simulink model "s1c"  (Simulink 2.00)
settings: Solver=ode113  StartTime=0.0  StopTime=tstop  MaxStep=1e-2  RelTol=1e-5  AbsTol=1e-6
values from neighbouring files (symbols this model uses):
  Domega = 0    [P20HP.M]
  H = J*wbm*wbm/(2*Sb)    (= 3.33396824273)    [P20HP.M]
  Psidso = 0    [M1C.M]    (also in M1O.M; M3.M)
  Psipdro = 0    [M1C.M]    (also in M1O.M; M3.M)
  Psipqro = 0    [M1C.M]    (also in M1O.M; M3.M)
  Psiqso = 0    [M1C.M]    (also in M1O.M; M3.M)
  rpr = 0.0764    [P20HP.M]
  rs = 0.1062    [P20HP.M]
  smaxt = rpr/rpr1    [M1C.M]    (also in M1O.M)
  speed_wref = [0 0.5 0.5 -0.5 -0.5 0]    [M1C.M]    (also in M1O.M = [0 1 1]; M3.M = [0 wbm/2 wbm/2 -wbm/2 -wbm/2 0])
  Tfactor = (3*P)/(4*wb)    (= 0.00795774715459)    [P20HP.M]
  time_tmech = [0 4]    [M1C.M]    (also in M1O.M = [0 0.75 0.75 1.0 1.0 1.25 1.25 1.5 1.5 2]; M3.M = [0 tstop])
  time_wref = [0 0.25 0.5 1.0 1.25 1.5]    [M1C.M]    (also in M1O.M = [0 0.5 4]; M3.M)
  tmech_tmech = [0 0]    [M1C.M]    (also in M1O.M = [0 0 -Trated -Trated -Trated/2 -Trated/2 -Trated -Trated 0 0; M3.M)
  vrms_vf = vrms    [M1C.M]    (also in M1O.M)
  wb = 2*pi*frated    (= 376.991118431)    [P20HP.M]
  we_vf = w    [M1C.M]    (also in M1O.M)
  wrbywbo = 0    [M1C.M]    (also in M1O.M; M3.M)
  xls = (we/wb)*xls    [M1C.M]    (also in M1O.M; M3.M; P20HP.M = 0.2145)
  xM = 1/(1/xm + 1/xls + 1/xplr)    [M1C.M]    (also in M1O.M; M3.M; P20HP.M = 0.105313916498)
  xplr = (we/wb)*xplr    [M1C.M]    (also in M1O.M; M3.M; P20HP.M = 0.2145)
  Zb = Vrated*Vrated/Sb    (= 3.24396782842)    [P20HP.M]
settings Model: MaxOrder=3  SaveTime=off  SaveOutput=off  ConsistencyChecking=off

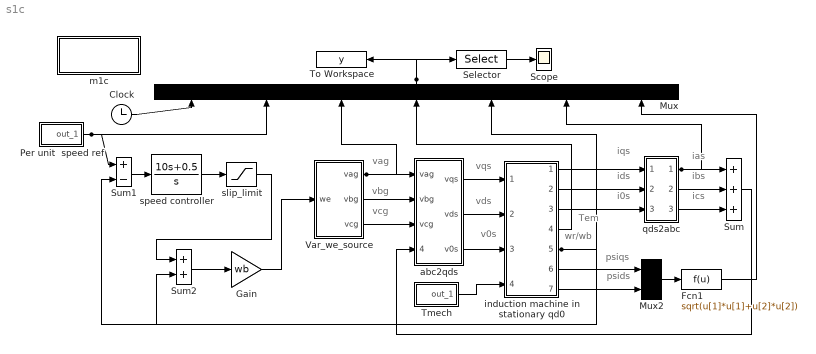
== system s1c ==
  note: wr/wb
  note: vcg
  note: vbg
  note: vag
  note: v0s
  note: vqs
  note: vds
  note: psiqs
  note: psids
  note: Tem
  note: i0s
  note: iqs
  note: ids
  note: ibs
  note: ias
  note: ics
  Clock : Clock
      settings: DeleteFcn=simclock BlockIsBeingDestroyed  PostSaveFcn=simclock Save
  Fcn1 : Fcn  Expr=sqrt(u[1]*u[1]+u[2]*u[2])
  Gain : Gain  Gain=wb
  m1c : Subsystem
      settings: OpenFcn=m1c
      mask Type: Masked block of m1c.m
      mask Help: Uses m1c.m to initialize and plot
      mask Display: disp('Initialize\nand plot')
  Mux : Mux  Orientation=up  Inputs=7
  Mux2 : Mux  Inputs=2
  "Per unit  speed ref " : Subsystem  mask(Repeating table){rep_seq_t=time_wref, rep_seq_y=speed_wref}
      mask prompts: rep_seq_t "Time values:"; rep_seq_y "Output values:"
      mask help: Repeating table.
      mask init:
      | period = max(rep_seq_t);
      mask Help: Repeats cycle given in table. Time values should be monotonically increasing.
      mask Display: plot([rep_seq_t,rep_seq_t+period,rep_seq_t+2*period,rep_seq_t(1)+3*period],[rep_seq_y,rep_seq_y,rep_seq_y,rep_seq_y(1)])
  Scope : Scope
      settings: TickLabels=on  TimeRange=2  YMin=-300  YMax=300  SaveToWorkspace=off  SaveName=ScopeData  LimitMaxRows=off
  Selector : Selector  Elements=[2 3 4 5 6 7]  InputPortWidth=7
  Sum : Sum  Inputs=+++
  Sum1 : Sum  Inputs=+-
  Sum2 : Sum  Inputs=++
  Tmech : Subsystem  mask(Repeating table){rep_seq_t=time_tmech, rep_seq_y=tmech_tmech}
      mask prompts: rep_seq_t "Time values:"; rep_seq_y "Output values:"
      mask help: Repeating table.
      mask init:
      | period = max(rep_seq_t);
      mask Help: Repeats cycle given in table. Time values should be monotonically increasing.
      mask Display: plot([rep_seq_t,rep_seq_t+period,rep_seq_t+2*period,rep_seq_t(1)+3*period],[rep_seq_y,rep_seq_y,rep_seq_y,rep_seq_y(1)])
  To Workspace : ToWorkspace  VariableName=y  SampleTime=0
      settings: Buffer=40000
  Var_we_source : Subsystem
  abc2qds : Subsystem
  induction machine in stationary qd0 : Subsystem
  qds2abc : Subsystem
  slip_limit : Saturate  UpperLimit=0.7*smaxt  LowerLimit=-0.7*smaxt
  speed controller : TransferFcn  Numerator=[10 0.5]  Denominator=[1 0]
  wires:
  abc2qds/3(v0s) -> induction machine in stationary qd0/3(in_v0s)
  Gain/1 -> Var_we_source/1(we)
  slip_limit/1 -> Sum2/1
  qds2abc/1(ias) -> Mux/6, Sum/1
  induction machine in stationary qd0/4(out_Tem) -> Mux/4
  Tmech/1(out_1) -> induction machine in stationary qd0/4(in_Tmech)
  Fcn1/1 -> Mux/7
  Var_we_source/1(vag) -> Mux/3, abc2qds/1(vag)
  "Per unit  speed ref "/1(out_1) -> Mux/2, Sum1/1
  Mux2/1 -> Fcn1/1
  induction machine in stationary qd0/7(out_psids) -> Mux2/2
  induction machine in stationary qd0/6(out_psiqs) -> Mux2/1
  speed controller/1 -> slip_limit/1
  induction machine in stationary qd0/5(out_wr/wb) -> Mux/5, Sum2/2, Sum1/2
  Sum2/1 -> Gain/1
  Sum1/1 -> speed controller/1
  induction machine in stationary qd0/3(out_i0s) -> qds2abc/3(i0s)
  induction machine in stationary qd0/2(out_ids) -> qds2abc/2(ids)
  induction machine in stationary qd0/1(out_iqs) -> qds2abc/1(iqs)
  abc2qds/2(vds) -> induction machine in stationary qd0/2(in_vds)
  Sum/1 -> abc2qds/4(ias+ibs+ics)
  qds2abc/3(ics) -> Sum/3
  qds2abc/2(ibs) -> Sum/2
  Var_we_source/3(vcg) -> abc2qds/3(vcg)
  Var_we_source/2(vbg) -> abc2qds/2(vbg)
  Clock/1 -> Mux/1
  abc2qds/1(vqs) -> induction machine in stationary qd0/1(in_vqs)
  Selector/1 -> Scope/1
  Mux/1 -> To Workspace/1, Selector/1

== system s1c/m1c ==
  note: Masked block of m1c.m
      | to initilialize simulation s1c.m
      | and to plot the results.

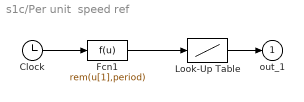
== system s1c/Per unit  speed ref  ==
  Clock : Clock
      settings: DeleteFcn=simclock BlockIsBeingDestroyed  PostSaveFcn=simclock Save
  Fcn1 : Fcn  Expr=rem(u[1],period)
  Look-Up Table : Lookup  InputValues=rep_seq_t  OutputValues=rep_seq_y
  out_1 : Outport  Port=1  InitialOutput=0
  wires:
  Fcn1/1 -> Look-Up Table/1
  Clock/1 -> Fcn1/1
  Look-Up Table/1 -> out_1/1

== system s1c/Tmech ==
  Clock : Clock
      settings: DeleteFcn=simclock BlockIsBeingDestroyed  PostSaveFcn=simclock Save
  Fcn1 : Fcn  Expr=rem(u[1],period)
  Look-Up Table : Lookup  InputValues=rep_seq_t  OutputValues=rep_seq_y
  out_1 : Outport  Port=1  InitialOutput=0
  wires:
  Fcn1/1 -> Look-Up Table/1
  Clock/1 -> Fcn1/1
  Look-Up Table/1 -> out_1/1

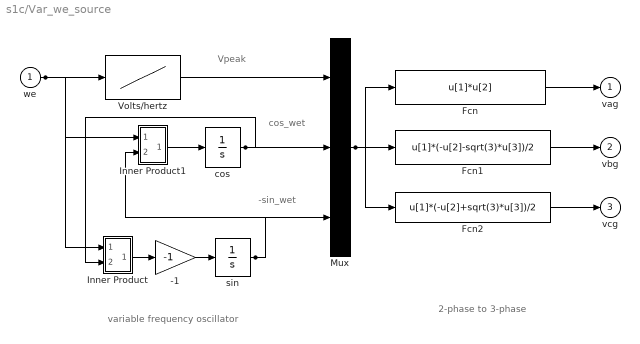
== system s1c/Var_we_source ==
  note: -sin_wet
  note: cos_wet
  note: variable frequency oscillator
  note: 2-phase to 3-phase
  note: Vpeak
  we : Inport  Port=1  PortWidth=-1  SampleTime=-1
  -1 : Gain  Gain=-1
  Fcn : Fcn  Expr=u[1]*u[2]
  Fcn1 : Fcn  Expr=u[1]*(-u[2]-sqrt(3)*u[3])/2
  Fcn2 : Fcn  Expr=u[1]*(-u[2]+sqrt(3)*u[3])/2
  Inner Product : Subsystem
      mask Type: Dot Product
      mask Description:
      | Inner (dot) product.
      | y=sum(u1.*u2)
      mask Help: Computes the inner (dot) product of the inputs: sum(u1.*u2).  The inputs are vectors of the same length. Output is a scalar.
      mask Display: disp('.\n')
  Inner Product1 : Subsystem
      mask Type: Dot Product
      mask Description:
      | Inner (dot) product.
      | y=sum(u1.*u2)
      mask Help: Computes the inner (dot) product of the inputs: sum(u1.*u2).  The inputs are vectors of the same length. Output is a scalar.
      mask Display: disp('.\n')
  Mux : Mux  Inputs=3
  Volts/hertz : Lookup  InputValues=we_vf  OutputValues=vrms_vf
  cos : Integrator  ExternalReset=none  InitialConditionSource=internal  InitialCondition=1  LimitOutput=off  UpperSaturationLimit=inf  LowerSaturationLimit=-inf  ShowSaturationPort=off  ShowStatePort=off  AbsoluteTolerance=auto
  sin : Integrator  ExternalReset=none  InitialConditionSource=internal  InitialCondition=0  LimitOutput=off  UpperSaturationLimit=inf  LowerSaturationLimit=-inf  ShowSaturationPort=off  ShowStatePort=off  AbsoluteTolerance=auto
  vag : Outport  Port=1  InitialOutput=0
  vbg : Outport  Port=2  InitialOutput=0
  vcg : Outport  Port=3  InitialOutput=0
  wires:
  Volts/hertz/1 -> Mux/1
  we/1 -> Volts/hertz/1, Inner Product/1(in_1), Inner Product1/1(in_1)
  Mux/1 -> Fcn2/1, Fcn1/1, Fcn/1
  Fcn2/1 -> vcg/1
  Fcn1/1 -> vbg/1
  Fcn/1 -> vag/1
  sin/1 -> Mux/3, Inner Product1/2(in_2)
  cos/1 -> Mux/2, Inner Product/2(in_2)
  Inner Product1/1(out_1) -> cos/1
  Inner Product/1(out_1) -> -1/1
  -1/1 -> sin/1

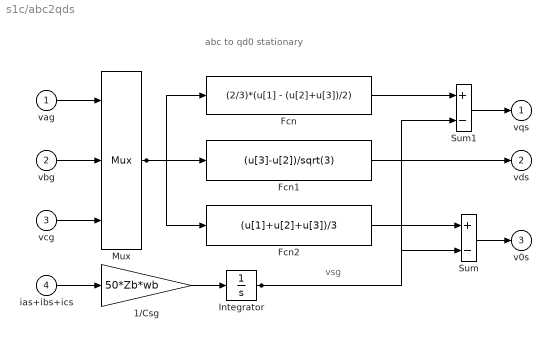
== system s1c/abc2qds ==
  note: vsg
  note: abc to qd0 stationary
  vag : Inport  Port=1  PortWidth=-1  SampleTime=-1
  vbg : Inport  Port=2  PortWidth=-1  SampleTime=-1
  vcg : Inport  Port=3  PortWidth=-1  SampleTime=-1
  ias+ibs+ics : Inport  Port=4  PortWidth=-1  SampleTime=-1
  1/Csg : Gain  Gain=50*Zb*wb
  Fcn : Fcn  Expr=(2/3)*(u[1] - (u[2]+u[3])/2)
  Fcn1 : Fcn  Expr=(u[3]-u[2])/sqrt(3)
  Fcn2 : Fcn  Expr=(u[1]+u[2]+u[3])/3
  Integrator : Integrator  ExternalReset=none  InitialConditionSource=internal  InitialCondition=0  LimitOutput=off  UpperSaturationLimit=inf  LowerSaturationLimit=-inf  ShowSaturationPort=off  ShowStatePort=off  AbsoluteTolerance=auto
  Mux : Mux  Inputs=3
  Sum : Sum  Inputs=+-
  Sum1 : Sum  Inputs=+-
  vqs : Outport  Port=1  InitialOutput=0
  vds : Outport  Port=2  InitialOutput=0
  v0s : Outport  Port=3  InitialOutput=0
  wires:
  Integrator/1 -> Sum1/2, Sum/2
  Sum1/1 -> vqs/1
  Fcn/1 -> Sum1/1
  1/Csg/1 -> Integrator/1
  Fcn2/1 -> Sum/1
  Sum/1 -> v0s/1
  Fcn1/1 -> vds/1
  Mux/1 -> Fcn2/1, Fcn/1, Fcn1/1
  vcg/1 -> Mux/3
  vbg/1 -> Mux/2
  vag/1 -> Mux/1
  ias+ibs+ics/1 -> 1/Csg/1

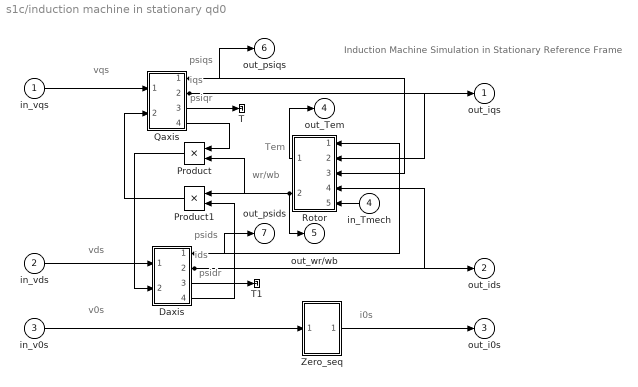
== system s1c/induction machine in stationary qd0 ==
  note: psiqs
  note: psids
  note: v0s
  note: i0s
  note: Tem
  note: wr/wb
  note: vds
  note: vqs
  note: ids
  note: psidr
  note: psiqr
  note: iqs
  note: Induction Machine Simulation
      |   in Stationary Reference Frame
  in_vqs : Inport  Port=1  PortWidth=-1  SampleTime=-1
  in_vds : Inport  Port=2  PortWidth=-1  SampleTime=-1
  in_v0s : Inport  Port=3  PortWidth=-1  SampleTime=-1
  in_Tmech : Inport  Orientation=left  Port=4  PortWidth=-1  SampleTime=-1
  Daxis : Subsystem
  Product : Product  Orientation=left  Inputs=2
  Product1 : Product  Orientation=left  Inputs=2
  Qaxis : Subsystem
  Rotor : Subsystem  Orientation=left
  T : Terminator
  T1 : Terminator
  Zero_seq : Subsystem
  out_iqs : Outport  Port=1  InitialOutput=0
  out_ids : Outport  Port=2  InitialOutput=0
  out_i0s : Outport  Port=3  InitialOutput=0
  out_Tem : Outport  Port=4  InitialOutput=0
  out_wr/wb : Outport  Port=5  InitialOutput=0
  out_psiqs : Outport  Port=6  InitialOutput=0
  out_psids : Outport  Port=7  InitialOutput=0
  wires:
  Daxis/3(out_idr') -> T1/1
  Qaxis/3(out_iqr') -> T/1
  Daxis/1(out_psids) -> out_psids/1, Rotor/1(in_psids)
  Qaxis/1(out_psiqs) -> out_psiqs/1, Rotor/3(in_psiqs)
  Daxis/2(out_ids) -> out_ids/1, Rotor/4(in_ids)
  Qaxis/2(out_iqs) -> out_iqs/1, Rotor/2(in_iqs)
  Zero_seq/1(out_i0s) -> out_i0s/1
  in_vds/1 -> Daxis/1(in_vds)
  in_v0s/1 -> Zero_seq/1(in_v0s)
  in_vqs/1 -> Qaxis/1(in_vqs)
  in_Tmech/1 -> Rotor/5(in_Tmech)
  Rotor/1(out_Tem) -> out_Tem/1
  Product1/1 -> Qaxis/2(in_(wr/wb)*psidr')
  Product/1 -> Daxis/2(in_(wr/wb)*psiqr')
  Rotor/2(out_wr/wb) -> out_wr/wb/1, Product/2, Product1/1
  Qaxis/4(out_psiqr') -> Product/1
  Daxis/4(out_psidr') -> Product1/2

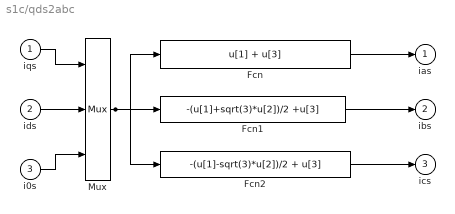
== system s1c/qds2abc ==
  iqs : Inport  Port=1  PortWidth=-1  SampleTime=-1
  ids : Inport  Port=2  PortWidth=-1  SampleTime=-1
  i0s : Inport  Port=3  PortWidth=-1  SampleTime=-1
  Fcn : Fcn  Expr=u[1] + u[3]
  Fcn1 : Fcn  Expr=-(u[1]+sqrt(3)*u[2])/2 +u[3]
  Fcn2 : Fcn  Expr=-(u[1]-sqrt(3)*u[2])/2 + u[3]
  Mux : Mux  Inputs=3
  ias : Outport  Port=1  InitialOutput=0
  ibs : Outport  Port=2  InitialOutput=0
  ics : Outport  Port=3  InitialOutput=0
  wires:
  Fcn2/1 -> ics/1
  Mux/1 -> Fcn2/1, Fcn/1, Fcn1/1
  Fcn/1 -> ias/1
  Fcn1/1 -> ibs/1
  i0s/1 -> Mux/3
  iqs/1 -> Mux/1
  ids/1 -> Mux/2

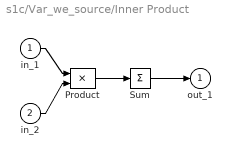
== system s1c/Var_we_source/Inner Product ==
  in_1 : Inport  Port=1  PortWidth=-1  SampleTime=-1
  in_2 : Inport  Port=2  PortWidth=-1  SampleTime=-1
  Product : Product  Inputs=2
  Sum : Sum  Inputs=+
  out_1 : Outport  Port=1  InitialOutput=0
  wires:
  Sum/1 -> out_1/1
  Product/1 -> Sum/1
  in_1/1 -> Product/1
  in_2/1 -> Product/2

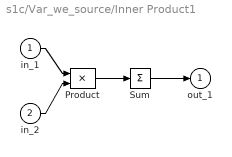
== system s1c/Var_we_source/Inner Product1 ==
  in_1 : Inport  Port=1  PortWidth=-1  SampleTime=-1
  in_2 : Inport  Port=2  PortWidth=-1  SampleTime=-1
  Product : Product  Inputs=2
  Sum : Sum  Inputs=+
  out_1 : Outport  Port=1  InitialOutput=0
  wires:
  Sum/1 -> out_1/1
  Product/1 -> Sum/1
  in_1/1 -> Product/1
  in_2/1 -> Product/2

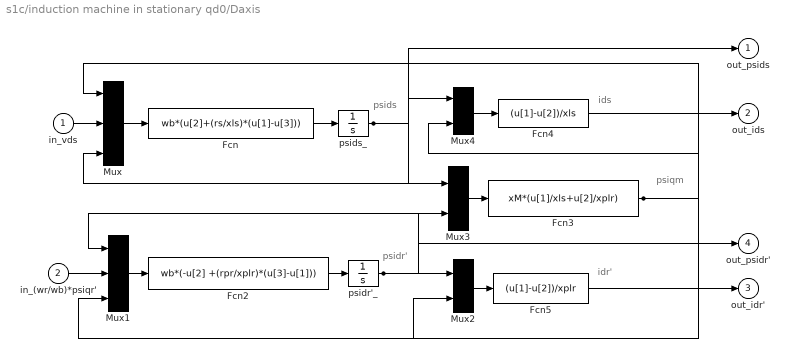
== system s1c/induction machine in stationary qd0/Daxis ==
  note: psidr'
  note: idr'
  note: psiqm
  note: psids
  note: ids
  in_vds : Inport  Port=1  PortWidth=-1  SampleTime=-1
  in_(wr/wb)*psiqr' : Inport  Port=2  PortWidth=-1  SampleTime=-1
  Fcn : Fcn  Expr=wb*(u[2]+(rs/xls)*(u[1]-u[3]))
  Fcn2 : Fcn  Expr=wb*(-u[2] +(rpr/xplr)*(u[3]-u[1]))
  Fcn3 : Fcn  Expr=xM*(u[1]/xls+u[2]/xplr)
  Fcn4 : Fcn  Expr=(u[1]-u[2])/xls
  Fcn5 : Fcn  Expr=(u[1]-u[2])/xplr
  Mux : Mux  Inputs=3
  Mux1 : Mux  Inputs=3
  Mux2 : Mux  Inputs=2
  Mux3 : Mux  Inputs=2
  Mux4 : Mux  Inputs=2
  psidr'_ : Integrator  ExternalReset=none  InitialConditionSource=internal  InitialCondition=Psipdro  LimitOutput=off  UpperSaturationLimit=inf  LowerSaturationLimit=-inf  ShowSaturationPort=off  ShowStatePort=off  AbsoluteTolerance=auto
  psids_ : Integrator  ExternalReset=none  InitialConditionSource=internal  InitialCondition=Psidso  LimitOutput=off  UpperSaturationLimit=inf  LowerSaturationLimit=-inf  ShowSaturationPort=off  ShowStatePort=off  AbsoluteTolerance=auto
  out_psids : Outport  Port=1  InitialOutput=0
  out_ids : Outport  Port=2  InitialOutput=0
  out_idr' : Outport  Port=3  InitialOutput=0
  out_psidr' : Outport  Port=4  InitialOutput=0
  wires:
  Fcn5/1 -> out_idr'/1
  in_(wr/wb)*psiqr'/1 -> Mux1/2
  in_vds/1 -> Mux/2
  Fcn4/1 -> out_ids/1
  Mux/1 -> Fcn/1
  Fcn/1 -> psids_/1
  Fcn2/1 -> psidr'_/1
  Mux3/1 -> Fcn3/1
  Mux4/1 -> Fcn4/1
  psids_/1 -> out_psids/1, Mux3/1, Mux4/1, Mux/3
  Fcn3/1 -> Mux4/2, Mux1/3, Mux/1, Mux2/2
  Mux1/1 -> Fcn2/1
  psidr'_/1 -> out_psidr'/1, Mux1/1, Mux3/2, Mux2/1
  Mux2/1 -> Fcn5/1

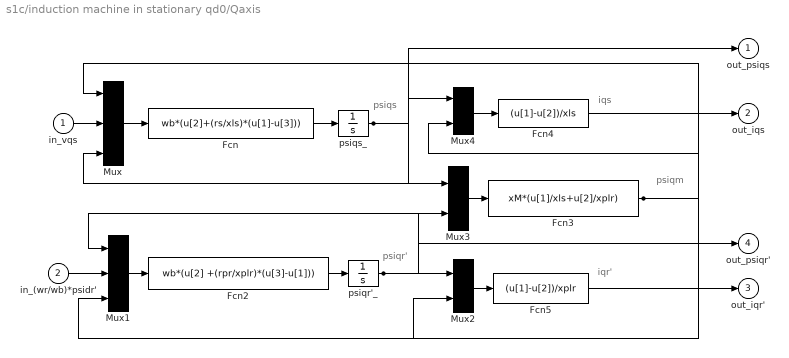
== system s1c/induction machine in stationary qd0/Qaxis ==
  note: psiqr'
  note: iqr'
  note: psiqm
  note: psiqs
  note: iqs
  in_vqs : Inport  Port=1  PortWidth=-1  SampleTime=-1
  in_(wr/wb)*psidr' : Inport  Port=2  PortWidth=-1  SampleTime=-1
  Fcn : Fcn  Expr=wb*(u[2]+(rs/xls)*(u[1]-u[3]))
  Fcn2 : Fcn  Expr=wb*(u[2] +(rpr/xplr)*(u[3]-u[1]))
  Fcn3 : Fcn  Expr=xM*(u[1]/xls+u[2]/xplr)
  Fcn4 : Fcn  Expr=(u[1]-u[2])/xls
  Fcn5 : Fcn  Expr=(u[1]-u[2])/xplr
  Mux : Mux  Inputs=3
  Mux1 : Mux  Inputs=3
  Mux2 : Mux  Inputs=2
  Mux3 : Mux  Inputs=2
  Mux4 : Mux  Inputs=2
  psiqr'_ : Integrator  ExternalReset=none  InitialConditionSource=internal  InitialCondition=Psipqro  LimitOutput=off  UpperSaturationLimit=inf  LowerSaturationLimit=-inf  ShowSaturationPort=off  ShowStatePort=off  AbsoluteTolerance=auto
  psiqs_ : Integrator  ExternalReset=none  InitialConditionSource=internal  InitialCondition=Psiqso  LimitOutput=off  UpperSaturationLimit=inf  LowerSaturationLimit=-inf  ShowSaturationPort=off  ShowStatePort=off  AbsoluteTolerance=auto
  out_psiqs : Outport  Port=1  InitialOutput=0
  out_iqs : Outport  Port=2  InitialOutput=0
  out_iqr' : Outport  Port=3  InitialOutput=0
  out_psiqr' : Outport  Port=4  InitialOutput=0
  wires:
  Fcn5/1 -> out_iqr'/1
  in_(wr/wb)*psidr'/1 -> Mux1/2
  in_vqs/1 -> Mux/2
  Fcn4/1 -> out_iqs/1
  Mux/1 -> Fcn/1
  Fcn/1 -> psiqs_/1
  Fcn2/1 -> psiqr'_/1
  Mux3/1 -> Fcn3/1
  Mux4/1 -> Fcn4/1
  psiqs_/1 -> out_psiqs/1, Mux3/1, Mux4/1, Mux/3
  Fcn3/1 -> Mux4/2, Mux1/3, Mux/1, Mux2/2
  Mux1/1 -> Fcn2/1
  psiqr'_/1 -> out_psiqr'/1, Mux1/1, Mux3/2, Mux2/1
  Mux2/1 -> Fcn5/1

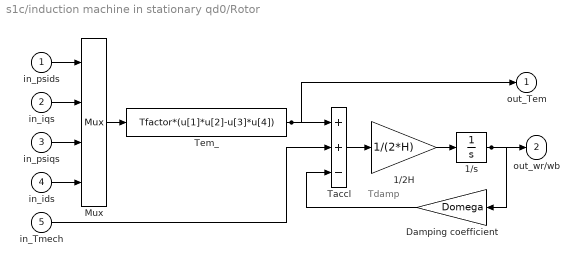
== system s1c/induction machine in stationary qd0/Rotor ==
  note: Tdamp
  in_psids : Inport  Port=1  PortWidth=-1  SampleTime=-1
  in_iqs : Inport  Port=2  PortWidth=-1  SampleTime=-1
  in_psiqs : Inport  Port=3  PortWidth=-1  SampleTime=-1
  in_ids : Inport  Port=4  PortWidth=-1  SampleTime=-1
  in_Tmech : Inport  Port=5  PortWidth=-1  SampleTime=-1
  1/2H : Gain  Gain=1/(2*H)
  1/s : Integrator  ExternalReset=none  InitialConditionSource=internal  InitialCondition=wrbywbo  LimitOutput=off  UpperSaturationLimit=inf  LowerSaturationLimit=-inf  ShowSaturationPort=off  ShowStatePort=off  AbsoluteTolerance=auto
  Damping coefficient : Gain  Orientation=left  Gain=Domega
  Mux : Mux  Inputs=4
  Taccl : Sum  Inputs=++-
  Tem_ : Fcn  Expr=Tfactor*(u[1]*u[2]-u[3]*u[4])
  out_Tem : Outport  Port=1  InitialOutput=0
  out_wr/wb : Outport  Port=2  InitialOutput=0
  wires:
  in_ids/1 -> Mux/4
  in_psiqs/1 -> Mux/3
  in_iqs/1 -> Mux/2
  in_psids/1 -> Mux/1
  Mux/1 -> Tem_/1
  Damping coefficient/1 -> Taccl/3
  1/s/1 -> Damping coefficient/1, out_wr/wb/1
  Tem_/1 -> out_Tem/1, Taccl/1
  1/2H/1 -> 1/s/1
  Taccl/1 -> 1/2H/1
  in_Tmech/1 -> Taccl/2

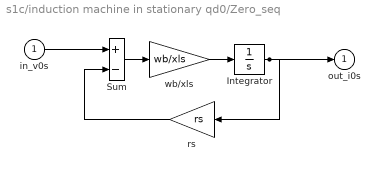
== system s1c/induction machine in stationary qd0/Zero_seq ==
  in_v0s : Inport  Port=1  PortWidth=-1  SampleTime=-1
  Integrator : Integrator  ExternalReset=none  InitialConditionSource=internal  InitialCondition=0  LimitOutput=off  UpperSaturationLimit=inf  LowerSaturationLimit=-inf  ShowSaturationPort=off  ShowStatePort=off  AbsoluteTolerance=auto
  Sum : Sum  Inputs=+-
  rs : Gain  Orientation=left  Gain=rs
  wb/xls : Gain  Gain=wb/xls
  out_i0s : Outport  Port=1  InitialOutput=0
  wires:
  Integrator/1 -> out_i0s/1, rs/1
  in_v0s/1 -> Sum/1
  wb/xls/1 -> Integrator/1
  Sum/1 -> wb/xls/1
  rs/1 -> Sum/2
